simulink model "FIR_filter"  (R2022b)
settings: Solver=VariableStepAuto  StartTime=0.0  StopTime=500  RelTol=1e-3
undefined symbols (not defined in the file): chirp, NTaps, Numerator1, Numerator2, T
libraries: simulink x3, simulink_need_slupdate x2, dspsrcs4 x1
settings Model: Creator=ASUS.PIESC  LastModifiedBy=ASUS.PIESC

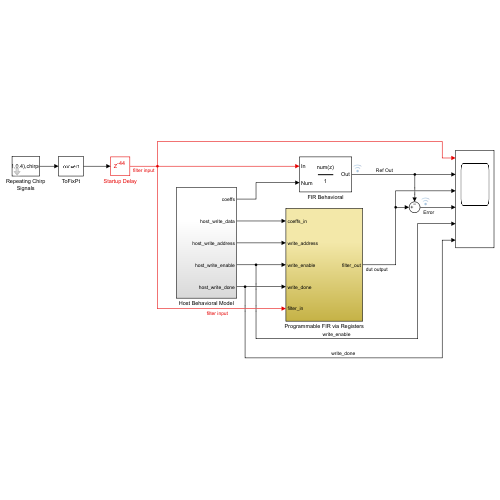
[thumbnail: Simulink's stored preview of the top-level diagram]
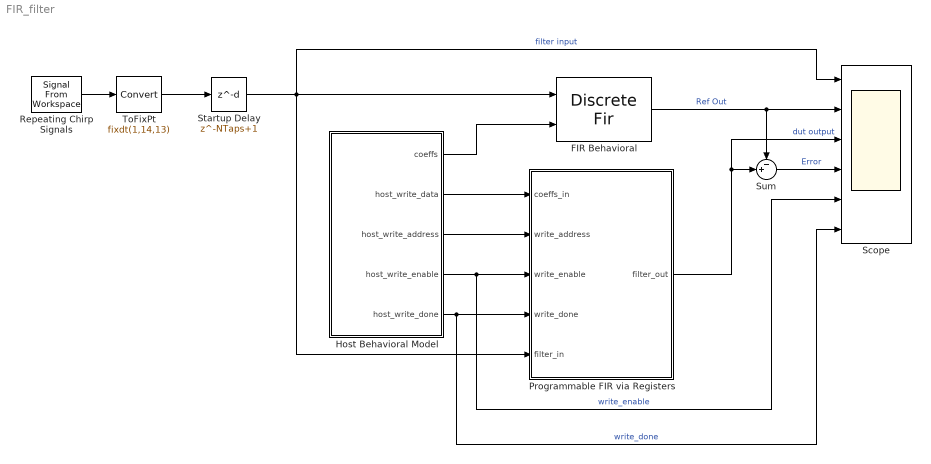
== system FIR_filter ==
  FIR Behavioral : DiscreteFir  CoefSource=Input port  Coefficients=Numerator2  InputProcessing=Columns as channels (frame based)  CoefDataTypeStr=fixdt(1,14,13)  ProductDataTypeStr=fixdt(1,29,29)  AccumDataTypeStr=fixdt(1,31,29)  OutDataTypeStr=fixdt(1,15,13)
      settings: InputPortMap=u0,u1
  Host Behavioral Model : Subsystem
  Programmable FIR via Registers : Subsystem
  Repeating Chirp Signals : dspsrcs4/Signal From Workspace  X=[chirp(0:T-1,0,T-1,0.4),chirp(0:T-1,0,T-1,0.4)]  Ts=1  nsamps=1  OutputAfterFinalValue=Setting to zero  ignoreOrWarnInputAndFrameLengths=off  OutputFrames=on
  Scope : Scope  NumInputPorts=6
  Startup Delay : Delay  DelayLength=NTaps+1
  Sum : Sum  Inputs=-+|
  ToFixPt : DataTypeConversion  OutDataTypeStr=fixdt(1,14,13)  RndMeth=Nearest
  wires:
  Host Behavioral Model/3(host_write_address) -> Programmable FIR via Registers/2(write_address)
  ToFixPt/1 -> Startup Delay/1
  Repeating Chirp Signals/1 -> ToFixPt/1
  Startup Delay/1 -> FIR Behavioral/1, Scope/1, Programmable FIR via Registers/5(filter_in)  "filter input"
  Host Behavioral Model/4(host_write_enable) -> Programmable FIR via Registers/3(write_enable), Scope/5  "write_enable"
  Host Behavioral Model/1(coeffs) -> FIR Behavioral/2
  FIR Behavioral/1 -> Scope/2, Sum/1  "Ref Out"
  Host Behavioral Model/2(host_write_data) -> Programmable FIR via Registers/1(coeffs_in)
  Programmable FIR via Registers/1(filter_out) -> Scope/3, Sum/2  "dut output"
  Host Behavioral Model/5(host_write_done) -> Programmable FIR via Registers/4(write_done), Scope/6  "write_done"
  Sum/1 -> Scope/4  "Error"

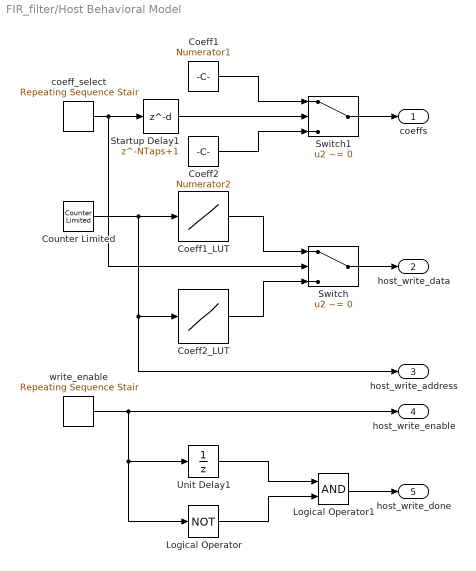
== system FIR_filter/Host Behavioral Model ==
  Coeff1 : Constant  Value=Numerator1  OutDataTypeStr=fixdt(1,14,13)  SampleTime=1
  Coeff1_LUT : Lookup  InputValues=[0:NTaps-1]  Table=Numerator1  LookUpMeth=Use Input Nearest  OutDataTypeStr=fixdt(1,14,13)  SaturateOnIntegerOverflow=off
  Coeff2 : Constant  Value=Numerator2  OutDataTypeStr=fixdt(1,14,13)  SampleTime=1
  Coeff2_LUT : Lookup  InputValues=[0:NTaps-1]  Table=Numerator2  LookUpMeth=Use Input Nearest  OutDataTypeStr=fixdt(1,14,13)  SaturateOnIntegerOverflow=off
  Counter Limited : simulink/Sources/Counter Limited  uplimit=NTaps-1  tsamp=-1
  Logical Operator : Logic  Operator=NOT  AllPortsSameDT=off  OutDataTypeStr=boolean
  Logical Operator1 : Logic  AllPortsSameDT=off  OutDataTypeStr=boolean
  Startup Delay1 : Delay  DelayLength=NTaps+1
  Switch : Switch  Criteria=u2 ~= 0  SaturateOnIntegerOverflow=off  InputSameDT=off
  Switch1 : Switch  Criteria=u2 ~= 0  SaturateOnIntegerOverflow=off  InputSameDT=off
  Unit Delay1 : UnitDelay  SampleTime=-1  HasFrameUpgradeWarning=on
  coeff_select : simulink/Sources/Repeating Sequence Stair  OutValues=[ones(T,1);zeros(T,1)]  tsamp=-1  OutMin=[]  OutMax=[]  OutDataTypeStr=fixdt('boolean')  OutputDataTypeScalingMode=Specify via dialog  OutDataType=fixdt('boolean')  ConRadixGroup=Best Precision: Vector-wise  OutScaling=[]
  write_enable : simulink/Sources/Repeating Sequence Stair  OutValues=[ones(NTaps,1); zeros(T-NTaps,1)]  tsamp=-1  OutMin=[]  OutMax=[]  OutDataTypeStr=fixdt('boolean')  OutputDataTypeScalingMode=Specify via dialog  OutDataType=fixdt('boolean')  ConRadixGroup=Best Precision: Vector-wise  OutScaling=[]
  coeffs : Outport  VectorParamsAs1DForOutWhenUnconnected=off
  host_write_data : Outport  Port=2  VectorParamsAs1DForOutWhenUnconnected=off
  host_write_address : Outport  Port=3  VectorParamsAs1DForOutWhenUnconnected=off
  host_write_enable : Outport  Port=4  OutDataTypeStr=boolean  VectorParamsAs1DForOutWhenUnconnected=off
  host_write_done : Outport  Port=5  VectorParamsAs1DForOutWhenUnconnected=off
  wires:
  Counter Limited/1 -> Coeff1_LUT/1, Coeff2_LUT/1, host_write_address/1
  Coeff1_LUT/1 -> Switch/1
  Switch/1 -> host_write_data/1
  Coeff2_LUT/1 -> Switch/3
  Coeff1/1 -> Switch1/1
  Coeff2/1 -> Switch1/3
  coeff_select/1 -> Startup Delay1/1, Switch/2
  Switch1/1 -> coeffs/1
  Startup Delay1/1 -> Switch1/2
  Unit Delay1/1 -> Logical Operator1/1
  Logical Operator/1 -> Logical Operator1/2
  Logical Operator1/1 -> host_write_done/1
  write_enable/1 -> Logical Operator/1, Unit Delay1/1, host_write_enable/1

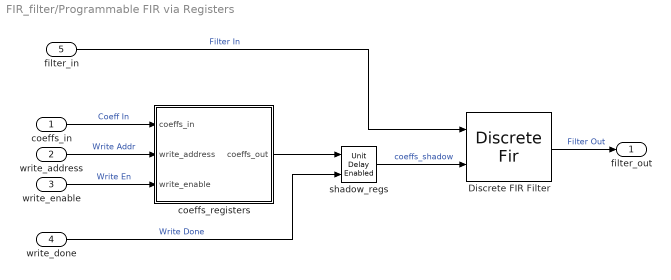
== system FIR_filter/Programmable FIR via Registers ==
  coeffs_in : Inport
  write_address : Inport  Port=2
  write_enable : Inport  Port=3
  write_done : Inport  Port=4
  filter_in : Inport  Port=5  PortDimensions=1
  Discrete FIR Filter : DiscreteFir  CoefSource=Input port  InputProcessing=Columns as channels (frame based)  ProductDataTypeStr=fixdt(1,29,29)  AccumDataTypeStr=fixdt(1,31,29)  OutDataTypeStr=fixdt(1,15,13)  SaturateOnIntegerOverflow=on
      settings: InputPortMap=u0,u1
  coeffs_registers : Subsystem  mask(Coefficients registers){numRegs=NTaps}
      mask prompts: numRegs "Number of registers"
      mask help: Store programmable coefficients in a register file, which is writable when 'write_enable' is true.
  shadow_regs : simulink_need_slupdate/Unit Delay Enabled  vinit=0.0  tsamp=-1
  filter_out : Outport  VectorParamsAs1DForOutWhenUnconnected=off
  wires:
  filter_in/1 -> Discrete FIR Filter/1  "Filter In"
  Discrete FIR Filter/1 -> filter_out/1  "Filter Out"
  coeffs_in/1 -> coeffs_registers/1(coeffs_in)  "Coeff In"
  write_address/1 -> coeffs_registers/2(write_address)  "Write Addr"
  write_enable/1 -> coeffs_registers/3(write_enable)  "Write En"
  write_done/1 -> shadow_regs/2  "Write Done"
  coeffs_registers/1(coeffs_out) -> shadow_regs/1
  shadow_regs/1 -> Discrete FIR Filter/2  "coeffs_shadow"

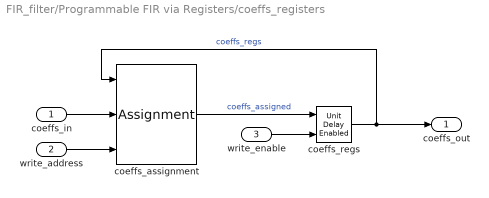
== system FIR_filter/Programmable FIR via Registers/coeffs_registers ==
  coeffs_in : Inport
  write_address : Inport  Port=2
  write_enable : Inport  Port=3
  coeffs_assignment : Assignment  IndexMode=Zero-based  IndexOptions=Index vector (port)  Indices=1  OutputSizes=[1 1]
  coeffs_regs : simulink_need_slupdate/Unit Delay Enabled  vinit=zeros(numRegs,1)  tsamp=-1
  coeffs_out : Outport  VectorParamsAs1DForOutWhenUnconnected=off
  wires:
  coeffs_assignment/1 -> coeffs_regs/1  "coeffs_assigned"
  coeffs_in/1 -> coeffs_assignment/2
  write_enable/1 -> coeffs_regs/2
  write_address/1 -> coeffs_assignment/3
  coeffs_regs/1 -> coeffs_out/1, coeffs_assignment/1  "coeffs_regs"
